simulink model "Question_3"  (R2018b)
settings: Solver=VariableStepAuto  StartTime=0.0  StopTime=10.0  RelTol=1e-3
libraries: cstblocks x4, RCTblocks x1
settings Model: Creator=auten  LastModifiedBy=auten

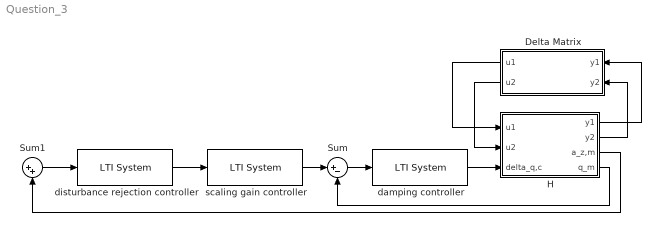
== system Question_3 ==
  Delta Matrix : Subsystem
  H : Subsystem
  Sum : Sum  Inputs=|+-
  Sum1 : Sum  Inputs=|++
  damping controller : cstblocks/LTI System  sys=K_q_value  IC=[]
  disturbance rejection controller : cstblocks/LTI System  sys=Kprime_dr  IC=[]
  scaling gain controller : cstblocks/LTI System  sys=K_sc_sim  IC=[]
  wires:
  H/2(y2) -> Delta Matrix/2(y2)
  Sum/1 -> damping controller/1
  disturbance rejection controller/1 -> scaling gain controller/1
  Delta Matrix/1(u1) -> H/1(u1)
  H/3(a_z,m) -> Sum1/2
  H/1(y1) -> Delta Matrix/1(y1)
  damping controller/1 -> H/3(delta_q,c)
  Sum1/1 -> disturbance rejection controller/1
  scaling gain controller/1 -> Sum/1
  Delta Matrix/2(u2) -> H/2(u2)
  H/4(q_m) -> Sum/2

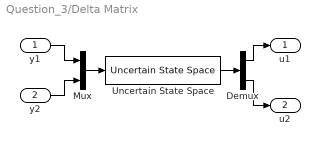
== system Question_3/Delta Matrix ==
  y1 : Inport
  y2 : Inport  Port=2
  Demux : Demux  Outputs=2
  Mux : Mux  Inputs=2
  Uncertain State Space : RCTblocks/Uncertain State Space  Tag=USS  USystem=Delta  UValue=Delta.Uncertainty  X0=[]  uX0=[]
      settings: SourceProductName=Robust Control Toolbox  SourceProductBaseCode=RC
  u1 : Outport
  u2 : Outport  Port=2
  wires:
  Mux/1 -> Uncertain State Space/1
  y1/1 -> Mux/1
  y2/1 -> Mux/2
  Demux/1 -> u1/1
  Demux/2 -> u2/1
  Uncertain State Space/1 -> Demux/1

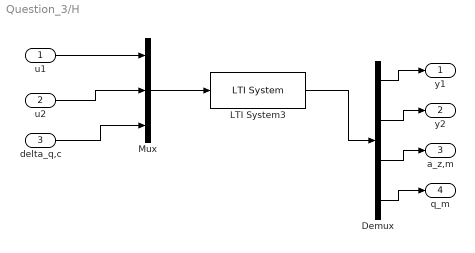
== system Question_3/H ==
  u1 : Inport
  u2 : Inport  Port=2
  delta_q,c : Inport  Port=3
  Demux : Demux
  LTI System3 : cstblocks/LTI System  sys=M  IC=[]
  Mux : Mux  Inputs=3
  y1 : Outport
  y2 : Outport  Port=2
  a_z,m : Outport  Port=3
  q_m : Outport  Port=4
  wires:
  u1/1 -> Mux/1
  u2/1 -> Mux/2
  delta_q,c/1 -> Mux/3
  Mux/1 -> LTI System3/1
  LTI System3/1 -> Demux/1
  Demux/1 -> y1/1
  Demux/2 -> y2/1
  Demux/3 -> a_z,m/1
  Demux/4 -> q_m/1
